simulink model "FrictionExp"  (R2017a)
settings: Solver=ode5  StartTime=0.0  StopTime=60  FixedStep=0.01  RelTol=1e-3
PreLoadFcn:
  | InvertedPendulumCtrlInit
values from neighbouring files (symbols this model uses):
  OffsetCart = 0    [PendulumParameters.m]
  OffsetPend = pi    (= 3.14159265359)    [PendulumParameters.m]
  ResCartEnc = 0.235 / 4096    (= 5.7373046875e-05)    [PendulumParameters.m]
  ResPendEnc = 2 * pi / 4096    (= 0.00153398078789)    [PendulumParameters.m]
  Ts = 0.01    [PendulumParameters.m]
  x0 = [0; 0; pi; 0]    [InvertedPendulumSimCtrlInit.m]
undefined symbols (not defined in the file): RTDAC4PCIBaseAddress
libraries: simulink x1
settings Model: SimulationMode=external  ExtModeTrigDuration=12000  ExtModeTrigLevel=0.400000  Creator=jims  LastModifiedBy=Pendulum
settings DataIOCC: SaveFormat=Array  SaveOutput=off  SignalLogging=off  DSMLogging=off  SaveTime=off  SignalLoggingName=sigsOut
settings OptimizationCC: DefaultParameterBehavior=Inlined  InlineInvariantSignals=on  EfficientFloat2IntCast=on  SimCompilerOptimization=on
settings DebuggingCC: SaveWithParameterizedLinksMsg=none  IntegerOverflowMsg=none  UniqueDataStoreMsg=error  AssertControl=DisableAll  StrictBusMsg=ErrorOnBusTreatedAsVector  SFUnexpectedBacktrackingDiag=warning  SFNoUnconditionalDefaultTransitionDiag=warning  SFExecutionAtInitializationDiag=none  IntegerSaturationMsg=none
settings ModelReferenceCC: PropagateSignalLabelsOutOfModel=off
settings SFSimCC: SimParseCustomCode=off
settings RTWCC: SystemTargetFile=sldrt.tlc  TemplateMakefile=sldrt.tmf  Description=Simulink Desktop Real-Time  RTWCompilerOptimization=on
settings CodeAppCC: MaxIdLength=95
settings SimulinkDesktopRealTimeCC: TargetPreCompLibLocation=C:\Program Files\MATLAB\R2017a\toolbox\sldrt\lib\win64  TargetLangStandard=C89/C90 (ANSI)  SupportVariableSizeSignals=off
settings ConfigComp: CovMetricSettings=dw  CovHtmlReporting=on  CovSaveCumulativeToWorkspaceVar=on  CovSaveSingleToWorkspaceVar=on  CovExternalEMLEnable=off  CovSFcnEnable=off

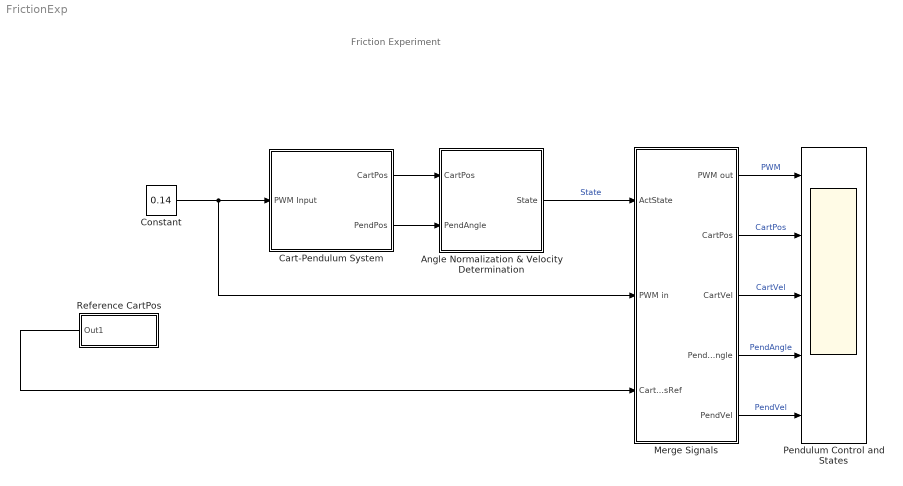
== system FrictionExp ==
  note: Friction Experiment
  Angle Normalization & Velocity Determination : Subsystem
  Cart-Pendulum System : Subsystem  mask(Cart-Pendulum System){BaseAddress=RTDAC4PCIBaseAddress(-1,-1)}
      mask prompts: BaseAddress "Base Address:"
      mask help: Interface to Cart-Pendulum System
      mask Display:
      | plot( [0.725 0.725], [1.15 0.375]); % pendulum arm
      | plot(0.725+0.05*sin([0:0.5:7]), 0.325+0.05*cos([0:0.5:7])); % pendulum load mass
      | plot([-0.2], [-0.2]);
      | plot([1.9], [1.7]);
      | plot([0.1 1.4], [1.09 1.09]); % upper rail
      | plot([0.1 1.4], [1.07 1.07]); % upper rail
      | plot([0.65 0.8], [1.1 1.1]); % cart bottom
      | plot([0.65 0.8], [1.2 1.2]); % cart top
      | plot([0.65 0.65], [1.2 1.1]); % cart left
      | plot([0.8 0.8], [1.1 1.2]); % cart right
      | port_label('input', 1, 'PWM');
      | port_label('output', 1, 'CartPos');
      | port_label('output', 2, 'PendAngle');
  Constant : Constant  Value=0.14
  Merge Signals : Subsystem
  Pendulum Control and States : Scope  NumInputPorts=5
  Reference CartPos : Subsystem  mask{Sine=off, Square=on, Sawtooth=off, Amplitude=0, Frequency=0.05}
      mask Display: disp('Generator')
  wires:
  Merge Signals/2(CartPos) -> Pendulum Control and States/2  "CartPos"
  Merge Signals/3(CartVel) -> Pendulum Control and States/3  "CartVel"
  Merge Signals/4(PendAngle) -> Pendulum Control and States/4  "PendAngle"
  Merge Signals/5(PendVel) -> Pendulum Control and States/5  "PendVel"
  Reference CartPos/1(Out1) -> Merge Signals/3(CartPosRef)
  Constant/1 -> Cart-Pendulum System/1(PWM Input), Merge Signals/2(PWM in)
  Cart-Pendulum System/2(PendPos) -> Angle Normalization & Velocity Determination/2(PendAngle)
  Angle Normalization & Velocity Determination/1(State) -> Merge Signals/1(ActState)  "State"
  Merge Signals/1(PWM out) -> Pendulum Control and States/1  "PWM"
  Cart-Pendulum System/1(CartPos) -> Angle Normalization & Velocity Determination/1(CartPos)

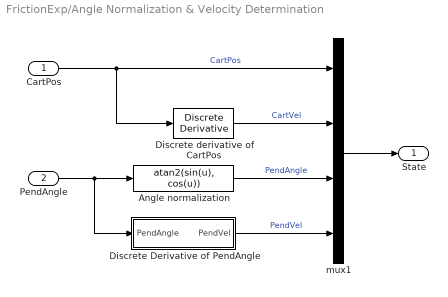
== system FrictionExp/Angle Normalization & Velocity Determination ==
  CartPos : Inport
  PendAngle : Inport  Port=2
  Angle normalization : Fcn  Expr=atan2(sin(u), cos(u))
  Discrete Derivative of PendAngle : Subsystem
  Discrete derivative of CartPos : simulink/Discrete/Discrete Derivative  gainval=1.0  ICPrevScaledInput=x0(1)/Ts  InputProcessing=Inherited  OutMin=[]  OutMax=[]  OutDataType=sfix(16)  OutScaling=2^-10  DoSatur=off
  mux1 : Mux
  State : Outport
  wires:
  Discrete Derivative of PendAngle/1(PendVel) -> mux1/4  "PendVel"
  Angle normalization/1 -> mux1/3  "PendAngle"
  Discrete derivative of CartPos/1 -> mux1/2  "CartVel"
  PendAngle/1 -> Discrete Derivative of PendAngle/1(PendAngle), Angle normalization/1
  mux1/1 -> State/1
  CartPos/1 -> mux1/1, Discrete derivative of CartPos/1  "CartPos"

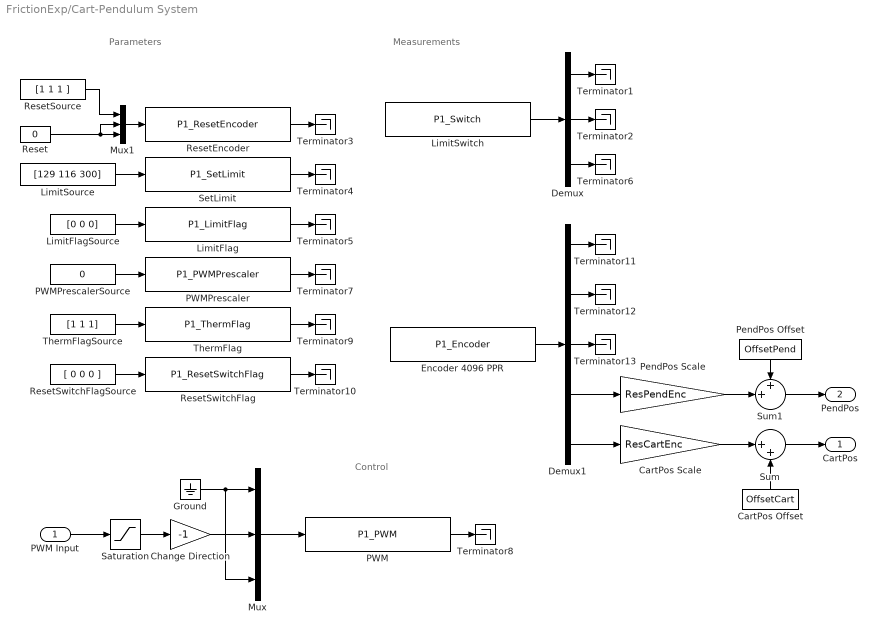
== system FrictionExp/Cart-Pendulum System ==
  note: Measurements
  note: Control
  note: Parameters
  PWM Input : Inport
  CartPos Offset : Constant  Value=OffsetCart
  CartPos Scale : Gain  Gain=ResCartEnc  OutDataTypeStr=Inherit: Same as input  ParamDataTypeStr=Inherit: Same as input
  Change Direction : Gain  Gain=-1  SaturateOnIntegerOverflow=on  OutDataTypeStr=Inherit: Same as input  ParamDataTypeStr=Inherit: Same as input
  Demux : Demux  Outputs=3
  Demux1 : Demux  Outputs=5
  Encoder 4096 PPR : S-Function  FunctionName=P1_Encoder  Parameters=BaseAddress, Ts  SFunctionDeploymentMode=off  EnableBusSupport=off
  Ground : Ground
  LimitFlag : S-Function  FunctionName=P1_LimitFlag  Parameters=BaseAddress, Ts  SFunctionDeploymentMode=off  EnableBusSupport=off
  LimitFlagSource : Constant  Value=[0 0 0]
  LimitSource : Constant  Value=[129 116 300]
  LimitSwitch : S-Function  FunctionName=P1_Switch  Parameters=BaseAddress, Ts  SFunctionDeploymentMode=off  EnableBusSupport=off
  Mux : Mux  Inputs=3
  Mux1 : Mux  Inputs=[3 1 1]
  PWM : S-Function  FunctionName=P1_PWM  Parameters=BaseAddress, Ts  SFunctionDeploymentMode=off  EnableBusSupport=off
  PWMPrescaler : S-Function  FunctionName=P1_PWMPrescaler  Parameters=BaseAddress, Ts  SFunctionDeploymentMode=off  EnableBusSupport=off
  PWMPrescalerSource : Constant  Value=0
  PendPos Offset : Constant  Value=OffsetPend
  PendPos Scale : Gain  Gain=ResPendEnc  OutDataTypeStr=Inherit: Same as input  ParamDataTypeStr=Inherit: Same as input
  Reset : Constant  Value=0
  ResetEncoder : S-Function  FunctionName=P1_ResetEncoder  Parameters=BaseAddress, Ts  SFunctionDeploymentMode=off  EnableBusSupport=off
  ResetSource : Constant  Value=[1 1 1 ]
  "ResetSwitchFlag " : S-Function  FunctionName=P1_ResetSwitchFlag  Parameters=BaseAddress, Ts  SFunctionDeploymentMode=off  EnableBusSupport=off
  ResetSwitchFlagSource : Constant  Value=[ 0 0 0 ]
  Saturation : Saturate
  SetLimit : S-Function  FunctionName=P1_SetLimit  Parameters=BaseAddress, Ts  SFunctionDeploymentMode=off  EnableBusSupport=off
  Sum : Sum  Inputs=|++  SaturateOnIntegerOverflow=on  InputSameDT=on  OutDataTypeStr=Inherit: Same as first input
  Sum1 : Sum  Inputs=++|  SaturateOnIntegerOverflow=on  InputSameDT=on  OutDataTypeStr=Inherit: Same as first input
  Terminator{1..13} (13 alike) : Terminator
  "ThermFlag " : S-Function  FunctionName=P1_ThermFlag  Parameters=BaseAddress, Ts  SFunctionDeploymentMode=off  EnableBusSupport=off
  ThermFlagSource : Constant  Value=[1 1 1]
  CartPos : Outport
  PendPos : Outport  Port=2
  wires:
  Demux1/1 -> Terminator11/1
  Demux1/2 -> Terminator12/1
  Demux1/3 -> Terminator13/1
  Demux1/4 -> PendPos Scale/1
  Demux1/5 -> CartPos Scale/1
  Demux/3 -> Terminator6/1
  Demux/2 -> Terminator2/1
  Demux/1 -> Terminator1/1
  LimitSwitch/1 -> Demux/1
  Ground/1 -> Mux/1, Mux/3
  ResetSwitchFlagSource/1 -> "ResetSwitchFlag "/1
  ThermFlagSource/1 -> "ThermFlag "/1
  PWMPrescalerSource/1 -> PWMPrescaler/1
  LimitFlagSource/1 -> LimitFlag/1
  LimitSource/1 -> SetLimit/1
  "ResetSwitchFlag "/1 -> Terminator10/1
  "ThermFlag "/1 -> Terminator9/1
  PWMPrescaler/1 -> Terminator7/1
  LimitFlag/1 -> Terminator5/1
  SetLimit/1 -> Terminator4/1
  ResetEncoder/1 -> Terminator3/1
  PWM/1 -> Terminator8/1
  Mux/1 -> PWM/1
  Encoder 4096 PPR/1 -> Demux1/1
  Mux1/1 -> ResetEncoder/1
  ResetSource/1 -> Mux1/1
  Change Direction/1 -> Mux/2
  PWM Input/1 -> Saturation/1
  PendPos Scale/1 -> Sum1/2
  PendPos Offset/1 -> Sum1/1
  Reset/1 -> Mux1/2, Mux1/3
  Saturation/1 -> Change Direction/1
  CartPos Offset/1 -> Sum/2
  CartPos Scale/1 -> Sum/1
  Sum/1 -> CartPos/1
  Sum1/1 -> PendPos/1

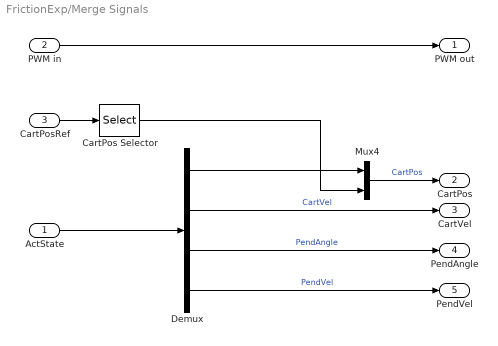
== system FrictionExp/Merge Signals ==
  ActState : Inport
  PWM in : Inport  Port=2
  CartPosRef : Inport  Port=3
  CartPos Selector : Selector  InputPortWidth=4  IndexOptions=Index vector (dialog)  Indices=[1]  OutputSizes=1
  Demux : Demux
  Mux4 : Mux  Inputs=2
  PWM out : Outport
  CartPos : Outport  Port=2
  CartVel : Outport  Port=3
  PendAngle : Outport  Port=4
  PendVel : Outport  Port=5
  wires:
  Mux4/1 -> CartPos/1  "CartPos"
  Demux/2 -> CartVel/1  "CartVel"
  Demux/3 -> PendAngle/1  "PendAngle"
  Demux/4 -> PendVel/1  "PendVel"
  Demux/1 -> Mux4/1
  CartPosRef/1 -> CartPos Selector/1
  ActState/1 -> Demux/1
  CartPos Selector/1 -> Mux4/2
  PWM in/1 -> PWM out/1

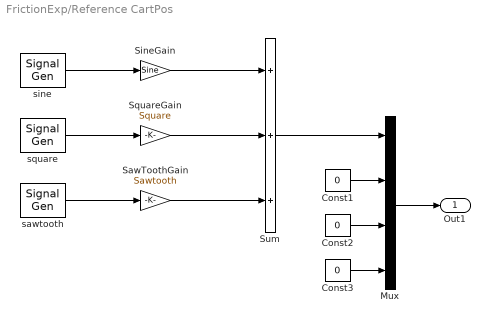
== system FrictionExp/Reference CartPos ==
  Const1 : Constant  Value=0
  Const2 : Constant  Value=0
  Const3 : Constant  Value=0
  Mux : Mux
  SawToothGain : Gain  Gain=Sawtooth  SaturateOnIntegerOverflow=on  OutDataTypeStr=Inherit: Same as input  ParamDataTypeStr=Inherit: Same as input
  SineGain : Gain  Gain=Sine  SaturateOnIntegerOverflow=on  OutDataTypeStr=Inherit: Same as input  ParamDataTypeStr=Inherit: Same as input
  SquareGain : Gain  Gain=Square  SaturateOnIntegerOverflow=on  OutDataTypeStr=Inherit: Same as input  ParamDataTypeStr=Inherit: Same as input
  Sum : Sum  Inputs=+++  SaturateOnIntegerOverflow=on  InputSameDT=on  OutDataTypeStr=Inherit: Same as first input
  sawtooth : SignalGenerator  WaveForm=sawtooth  Amplitude=Amplitude  Frequency=Frequency
  sine : SignalGenerator  Amplitude=Amplitude  Frequency=Frequency
  square : SignalGenerator  WaveForm=square  Amplitude=Amplitude  Frequency=Frequency
  Out1 : Outport
  wires:
  SawToothGain/1 -> Sum/3
  SquareGain/1 -> Sum/2
  SineGain/1 -> Sum/1
  sawtooth/1 -> SawToothGain/1
  square/1 -> SquareGain/1
  sine/1 -> SineGain/1
  Const2/1 -> Mux/3
  Const3/1 -> Mux/4
  Mux/1 -> Out1/1
  Const1/1 -> Mux/2
  Sum/1 -> Mux/1

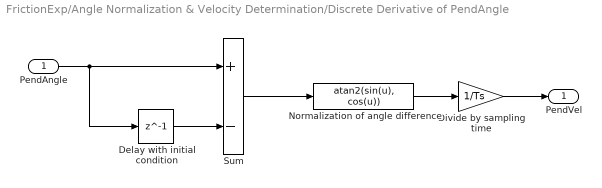
== system FrictionExp/Angle Normalization & Velocity Determination/Discrete Derivative of PendAngle ==
  PendAngle : Inport
  Delay with initial condition : Delay  DelayLength=1  InitialCondition=x0(3)
  Divide by sampling time : Gain  Gain=1/Ts
  Normalization of angle difference : Fcn  Expr=atan2(sin(u), cos(u))
  Sum : Sum  Inputs=+-
  PendVel : Outport
  wires:
  Sum/1 -> Normalization of angle difference/1
  Normalization of angle difference/1 -> Divide by sampling time/1
  Divide by sampling time/1 -> PendVel/1
  PendAngle/1 -> Delay with initial condition/1, Sum/1
  Delay with initial condition/1 -> Sum/2
